simulink model "main"  (R2020a)
settings: Solver=VariableStepAuto  StartTime=0.0  StopTime=10.0  RelTol=1e-3
settings Model: Creator=fsepcke  LastModifiedBy=fsepcke

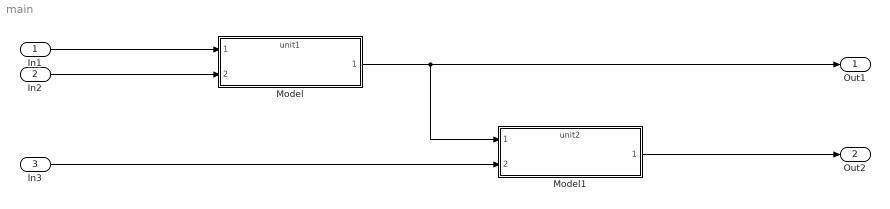
== system main ==
  In1 : Inport
  In2 : Inport  Port=2
  In3 : Inport  Port=3
  Model : ModelReference  ModelNameDialog=unit1  SimulationMode=Normal  ModelReferenceVersion=1.1
  Model1 : ModelReference  ModelNameDialog=unit2  SimulationMode=Normal  ModelReferenceVersion=1.1
  Out1 : Outport
  Out2 : Outport  Port=2
  wires:
  In1/1 -> Model/1
  In2/1 -> Model/2
  Model/1 -> Out1/1, Model1/1
  In3/1 -> Model1/2
  Model1/1 -> Out2/1
